simulink model "sch_pendule_etudiant"  (R2016a)
settings: Solver=ode45  StartTime=0.0  StopTime=10.0  RelTol=1e-3
values from neighbouring files (symbols this model uses):
  CH = struct()    [prg_pendule_etudiant.m]
settings Model: Creator=Zouhair  LastModifiedBy=hp
settings DataIOCC: LimitDataPoints=on  SaveFormat=Array
settings HardwareCC: ProdBitPerPointer=32  ProdLargestAtomicFloat=None  ProdIntDivRoundTo=Undefined  ProdEndianess=Unspecified  ProdWordSize=32  ProdHWDeviceType=32-bit Generic
settings ModelReferenceCC: PropagateSignalLabelsOutOfModel=off
settings ConfigComp: CovModelRefEnable=Off

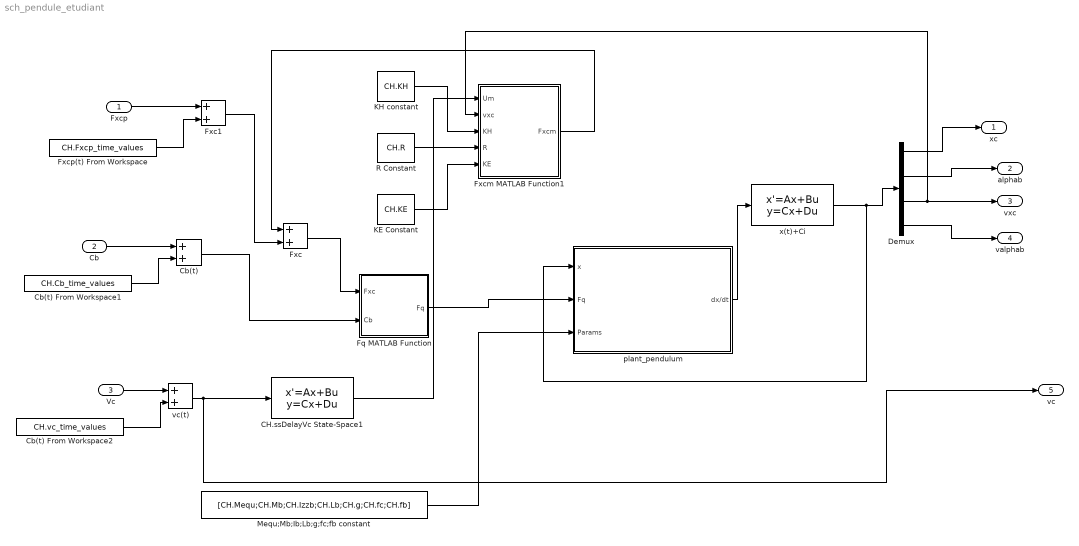
== system sch_pendule_etudiant ==
  Fxcp : Inport
  Cb : Inport  Port=2
  Vc : Inport  Port=3
  CH.ssDelayVc State-Space1 : StateSpace  A=CH.ssDelayVc.A  B=CH.ssDelayVc.B  C=CH.ssDelayVc.C  D=CH.ssDelayVc.D  X0=0
  Cb(t) : Sum
  Cb(t) From Workspace1 : FromWorkspace  VariableName=CH.Cb_time_values  SampleTime=0  OutputAfterFinalValue=Holding final value
  Cb(t) From Workspace2 : FromWorkspace  VariableName=CH.vc_time_values  SampleTime=0  OutputAfterFinalValue=Holding final value
  Demux : Demux
  Fq MATLAB Function : MATLAB Function  TreatAsAtomicUnit=on
  Fxc : Sum
  Fxc1 : Sum
  Fxcm MATLAB Function1 : MATLAB Function  TreatAsAtomicUnit=on
  Fxcp(t) From Workspace : FromWorkspace  VariableName=CH.Fxcp_time_values  SampleTime=0  OutputAfterFinalValue=Holding final value
  "KE Constant " : Constant  Value=CH.KE
  "KH constant " : Constant  Value=CH.KH
  Mequ;Mb;Ib;Lb;g;fc;fb constant : Constant  Value=[CH.Mequ;CH.Mb;CH.Izzb;CH.Lb;CH.g;CH.fc;CH.fb]
  R Constant : Constant  Value=CH.R
  plant_pendulum : Subsystem
  vc(t) : Sum
  x(t)+Ci : StateSpace  A=zeros(4,4)  B=eye(4,4)  C=eye(4,4)  D=zeros(4,4)  X0=[CH.xc_init;CH.alphab_init;CH.vxc_init;CH.valphab_init]
  xc : Outport
  alphab : Outport  Port=2
  vxc : Outport  Port=3
  valphab : Outport  Port=4
  vc : Outport  Port=5
  wires:
  Fxc/1 -> Fq MATLAB Function/1(Fxc)
  Cb(t)/1 -> Fq MATLAB Function/2(Cb)
  Fxcp/1 -> Fxc1/1
  Fxcp(t) From Workspace/1 -> Fxc1/2
  Fxc1/1 -> Fxc/2
  Cb/1 -> Cb(t)/1
  Cb(t) From Workspace1/1 -> Cb(t)/2
  Vc/1 -> vc(t)/1
  Cb(t) From Workspace2/1 -> vc(t)/2
  vc(t)/1 -> vc/1, CH.ssDelayVc State-Space1/1
  "KH constant "/1 -> Fxcm MATLAB Function1/3(KH)
  R Constant/1 -> Fxcm MATLAB Function1/4(R)
  "KE Constant "/1 -> Fxcm MATLAB Function1/5(KE)
  Fxcm MATLAB Function1/1(Fxcm) -> Fxc/1
  CH.ssDelayVc State-Space1/1 -> Fxcm MATLAB Function1/1(Um)
  Demux/1 -> xc/1
  Demux/2 -> alphab/1
  Demux/3 -> vxc/1, Fxcm MATLAB Function1/2(vxc)
  Demux/4 -> valphab/1
  Fq MATLAB Function/1(Fq) -> plant_pendulum/2(Fq)
  Mequ;Mb;Ib;Lb;g;fc;fb constant/1 -> plant_pendulum/3(Params)
  plant_pendulum/1(dx/dt) -> x(t)+Ci/1
  x(t)+Ci/1 -> Demux/1, plant_pendulum/1(x)

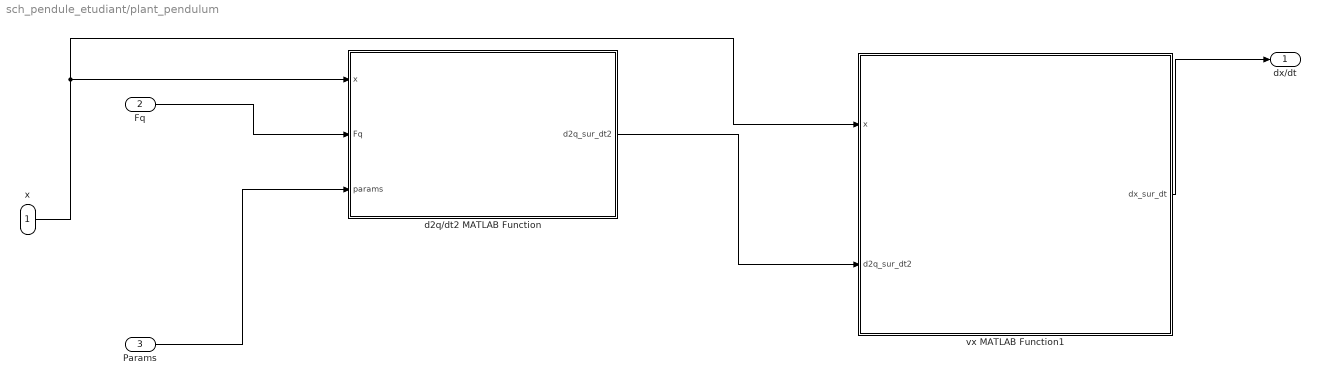
== system sch_pendule_etudiant/plant_pendulum ==
  x : Inport
  Fq : Inport  Port=2
  Params : Inport  Port=3
  d2q/dt2 MATLAB Function : MATLAB Function  TreatAsAtomicUnit=on
  vx MATLAB Function1 : MATLAB Function  TreatAsAtomicUnit=on
  dx/dt : Outport
  wires:
  x/1 -> vx MATLAB Function1/1(x), d2q/dt2 MATLAB Function/1(x)
  vx MATLAB Function1/1(dx_sur_dt) -> dx/dt/1
  d2q/dt2 MATLAB Function/1(d2q_sur_dt2) -> vx MATLAB Function1/2(d2q_sur_dt2)
  Fq/1 -> d2q/dt2 MATLAB Function/2(Fq)
  Params/1 -> d2q/dt2 MATLAB Function/3(params)

== matlab function sch_pendule_etudiant/plant_pendulum/vx MATLAB Function1 ==
  data: x input; dx_sur_dt output; d2q_sur_dt2 input
function dx_sur_dt = my_dx_sur_dt(x,d2q_sur_dt2)
dq_sur_dt=x(3:4,1);

dx_sur_dt =[dq_sur_dt;d2q_sur_dt2];

== matlab function sch_pendule_etudiant/plant_pendulum/d2q//dt2 MATLAB Function ==
  data: x input; d2q_sur_dt2 output; Fq input; params input
function d2q_sur_dt2 = clc_accq(x,Fq,params)
%[CH.Mequ;CH.Mb;CH.Ib;CH.Lb;CH.g;CH.fc;CH.fb]
xc=x(1);
alphab=x(2);
vxc=x(3);
valphab=x(4);
%2extraction desparemetres
Mequ=params(1);
Mb=params(2);
Ib=params(3);
Lb=params(4);
g=params(5);
fc=params(6);
fb=params(7);
%composant A
A11=Mequ+Mb;
A12=-Lb*Mb*sin(alphab);
A21=A12;
A22=Ib;
%composant H
H1=fc*vxc;
H2=fb*valphab+Mb*Lb*g*cos(alphab);
A=[A11 A12;A21 A22];
H=[H1;H2];
%pinv la pseudo inverse 
d2q_sur_dt2=pinv(A)*(Fq-H);

== matlab function sch_pendule_etudiant/Fq MATLAB Function ==
  data: Fxc input; Fq output; Cb input
function Fq = fcn(Fxc,Cb)


Fq = [Fxc;Cb];

== matlab function sch_pendule_etudiant/Fxcm MATLAB Function1 ==
  data: Um input; Fxcm output; vxc input; KH input; R input; KE input
function Fxcm = clc_moteur(Um,vxc,KH,R,KE)
%calcule de Fxcm
%Um=tension d'induit en volt
%U=tension de commande en volt
%Fxcm en Newton
%KH= gain du hacheur
%KE=coefficient du moteur 
%R=resistance d'induit du moteur
U=KH*Um;
e=KE*vxc;
I=(U-e)/R;
Fxcm = KE*I;
